simulink model "ball_and_plate"  (Simulink 7.6)
settings: Solver=ode45  StartTime=0.0  StopTime=20.0  RelTol=1e-3
undefined symbols (not defined in the file): magnitude
libraries: simulink x15
settings Model: Creator=Marco  LastModifiedBy=Marco

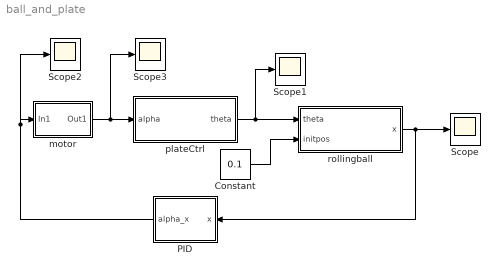
== system ball_and_plate ==
  Constant : Constant  Value=0.1
  PID : Subsystem
  Scope{,1..3} (4 alike) : Scope
      Scope settings: TimeRange=20  YMin=-2.5e+033  YMax=7e+033
      Scope2 settings: SaveName=ScopeData3
      Scope3 settings: SaveName=ScopeData4
  motor : Subsystem
  plateCtrl : Subsystem
  rollingball : Subsystem
  wires:
  plateCtrl/1(theta) -> rollingball/1(theta), Scope1/1
  rollingball/1(x) -> Scope/1, PID/1(x)
  Constant/1 -> rollingball/2(initpos)
  PID/1(alpha_x) -> motor/1(In1), Scope2/1
  motor/1(Out1) -> plateCtrl/1(alpha), Scope3/1

== system ball_and_plate/PID ==
  x : Inport
  controller : Subsystem
  alpha_x : Outport
  wires:
  controller/1(Out1) -> alpha_x/1
  x/1 -> controller/1(x)

== system ball_and_plate/motor ==
  In1 : Inport
  Rate Limiter : RateLimiter  RisingSlewLimit=7  FallingSlewLimit=-7  SampleTimeMode=inherited
  Out1 : Outport
  wires:
  In1/1 -> Rate Limiter/1
  Rate Limiter/1 -> Out1/1

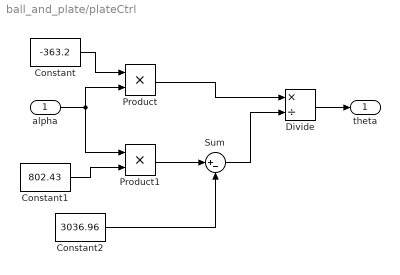
== system ball_and_plate/plateCtrl ==
  alpha : Inport
  Constant : Constant  Value=-363.2
  Constant1 : Constant  Value=802.43
  Constant2 : Constant  Value=3036.96
  Divide : Product  Inputs=*/
  Product : Product  RndMeth=Zero
  Product1 : Product  RndMeth=Zero
  Sum : Sum  Inputs=|+-
  theta : Outport
  wires:
  Constant/1 -> Product/1
  alpha/1 -> Product/2, Product1/1
  Constant1/1 -> Product1/2
  Product1/1 -> Sum/1
  Constant2/1 -> Sum/2
  Divide/1 -> theta/1
  Product/1 -> Divide/1
  Sum/1 -> Divide/2

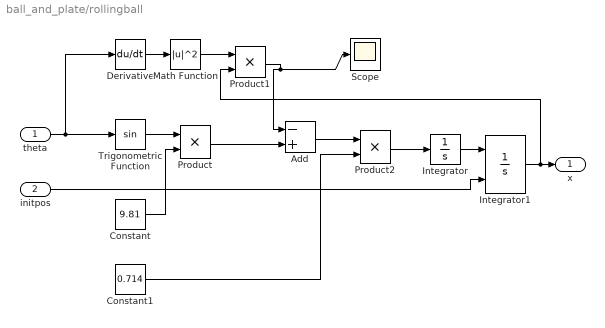
== system ball_and_plate/rollingball ==
  theta : Inport
  initpos : Inport  Port=2
  Add : Sum  Inputs=-+
  Constant : Constant  Value=9.81
  Constant1 : Constant  Value=0.714
  Derivative : Derivative
  Integrator : Integrator
  Integrator1 : Integrator  InitialConditionSource=external
  Math Function : Math  Operator=magnitude^2  SaturateOnIntegerOverflow=on
  Product : Product  RndMeth=Zero
  Product1 : Product  RndMeth=Zero
  Product2 : Product  RndMeth=Zero
  Scope : Scope
      settings: SaveName=ScopeData2
  Trigonometric Function : Trigonometry
  x : Outport
  wires:
  theta/1 -> Trigonometric Function/1, Derivative/1
  Trigonometric Function/1 -> Product/1
  Constant/1 -> Product/2
  Integrator/1 -> Integrator1/1
  Integrator1/1 -> Product1/2, x/1
  initpos/1 -> Integrator1/2
  Derivative/1 -> Math Function/1
  Math Function/1 -> Product1/1
  Product2/1 -> Integrator/1
  Constant1/1 -> Product2/2
  Add/1 -> Product2/1
  Product/1 -> Add/2
  Product1/1 -> Scope/1, Add/1

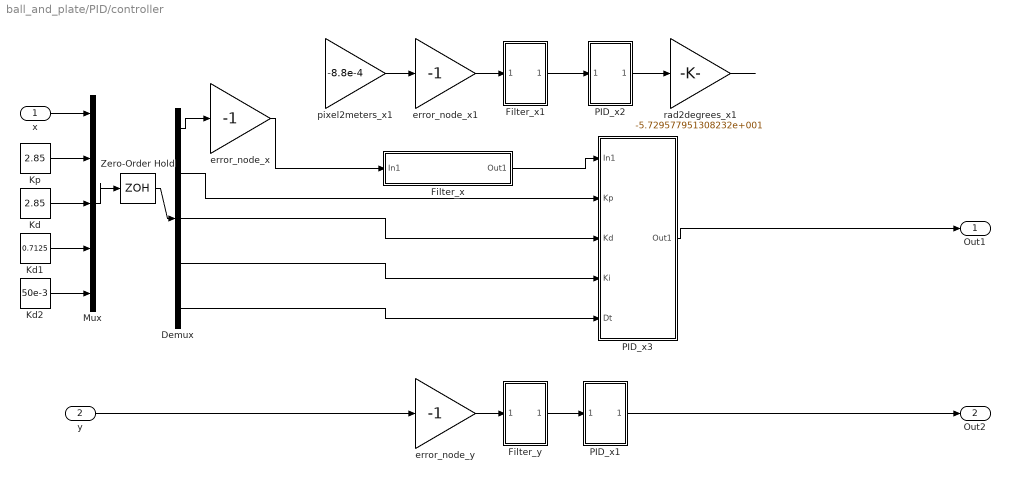
== system ball_and_plate/PID/controller ==
  x : Inport
  y : Inport  Port=2
  Demux : Demux  Outputs=5
  Filter_x : Subsystem
  Filter_x1 : Subsystem
  Filter_y : Subsystem
  Kd : Constant  Value=2.85  SampleTime=0
  Kd1 : Constant  Value=0.7125  SampleTime=0
  Kd2 : Constant  Value=50e-3  SampleTime=0
  Kp : Constant  Value=2.85  SampleTime=0
  Mux : Mux  Inputs=5
  PID_x1 : Subsystem
  PID_x2 : Subsystem
  PID_x3 : Subsystem
  Zero-Order Hold : ZeroOrderHold  SampleTime=50e-3
  error_node_x : Gain  Gain=-1
  error_node_x1 : Gain  Gain=-1
  error_node_y : Gain  Gain=-1  SampleTime=50e-3
  pixel2meters_x1 : Gain  Gain=-8.8e-4
  rad2degrees_x1 : Gain  Gain=-5.729577951308232e+001  SampleTime=50e-3
  Out1 : Outport
  Out2 : Outport  Port=2
  wires:
  PID_x1/1(Out1) -> Out2/1
  y/1 -> error_node_y/1
  Filter_x1/1(Out1) -> PID_x2/1(In1)
  rad2degrees_x1/1 -> ?
  error_node_x1/1 -> Filter_x1/1(In1)
  ? -> pixel2meters_x1/1
  pixel2meters_x1/1 -> error_node_x1/1
  PID_x2/1(Out1) -> rad2degrees_x1/1
  PID_x3/1(Out1) -> Out1/1
  error_node_y/1 -> Filter_y/1(In1)
  Filter_y/1(Out1) -> PID_x1/1(In1)
  error_node_x/1 -> Filter_x/1(In1)
  Filter_x/1(Out1) -> PID_x3/1(In1)
  x/1 -> Mux/1
  Mux/1 -> Zero-Order Hold/1
  Zero-Order Hold/1 -> Demux/1
  Demux/1 -> error_node_x/1
  Kd/1 -> Mux/3
  Kd1/1 -> Mux/4
  Demux/3 -> PID_x3/3(Kd)
  Demux/4 -> PID_x3/4(Ki)
  Kd2/1 -> Mux/5
  Demux/5 -> PID_x3/5(Dt)
  Kp/1 -> Mux/2
  Demux/2 -> PID_x3/2(Kp)

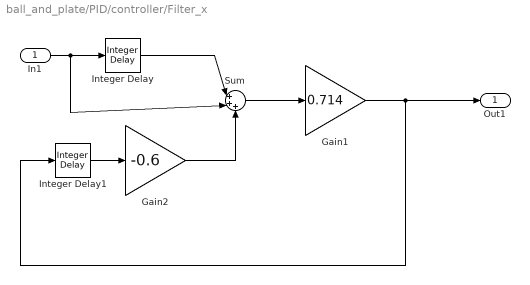
== system ball_and_plate/PID/controller/Filter_x ==
  In1 : Inport
  Gain1 : Gain  Gain=0.714
  Gain2 : Gain  Gain=-0.6
  Integer Delay : simulink/Discrete/Integer Delay  NumDelays=1  InputProcessing=Inherited  vinit=0.0  samptime=-1
  Integer Delay1 : simulink/Discrete/Integer Delay  NumDelays=1  InputProcessing=Inherited  vinit=0.0  samptime=-1
  Sum : Sum  Inputs=|+++
  Out1 : Outport
  wires:
  Sum/1 -> Gain1/1
  Gain1/1 -> Integer Delay1/1, Out1/1
  Integer Delay1/1 -> Gain2/1
  Integer Delay/1 -> Sum/1
  Gain2/1 -> Sum/3
  In1/1 -> Integer Delay/1, Sum/2

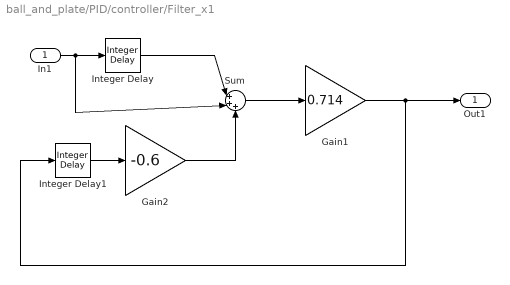
== system ball_and_plate/PID/controller/Filter_x1 ==
  In1 : Inport
  Gain1 : Gain  Gain=0.714  SampleTime=50e-3
  Gain2 : Gain  Gain=-0.6  SampleTime=50e-3
  Integer Delay : simulink/Discrete/Integer Delay  NumDelays=1  InputProcessing=Inherited  vinit=0.0  samptime=-1
  Integer Delay1 : simulink/Discrete/Integer Delay  NumDelays=1  InputProcessing=Inherited  vinit=0.0  samptime=50e-3
  Sum : Sum  Inputs=|+++  SampleTime=50e-3
  Out1 : Outport
  wires:
  In1/1 -> Integer Delay/1, Sum/2
  Sum/1 -> Gain1/1
  Gain1/1 -> Out1/1, Integer Delay1/1
  Integer Delay1/1 -> Gain2/1
  Integer Delay/1 -> Sum/1
  Gain2/1 -> Sum/3

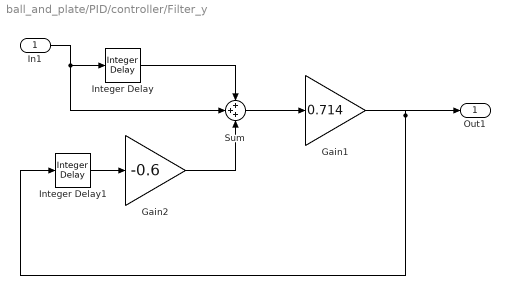
== system ball_and_plate/PID/controller/Filter_y ==
  In1 : Inport
  Gain1 : Gain  Gain=0.714  SampleTime=50e-3
  Gain2 : Gain  Gain=-0.6  SampleTime=50e-3
  Integer Delay : simulink/Discrete/Integer Delay  NumDelays=1  InputProcessing=Inherited  vinit=0.0  samptime=50e-3
  Integer Delay1 : simulink/Discrete/Integer Delay  NumDelays=1  InputProcessing=Inherited  vinit=0.0  samptime=50e-3
  Sum : Sum  Inputs=+++  SampleTime=50e-3
  Out1 : Outport
  wires:
  Integer Delay1/1 -> Gain2/1
  Gain1/1 -> Integer Delay1/1, Out1/1
  Sum/1 -> Gain1/1
  Integer Delay/1 -> Sum/1
  In1/1 -> Integer Delay/1, Sum/2
  Gain2/1 -> Sum/3

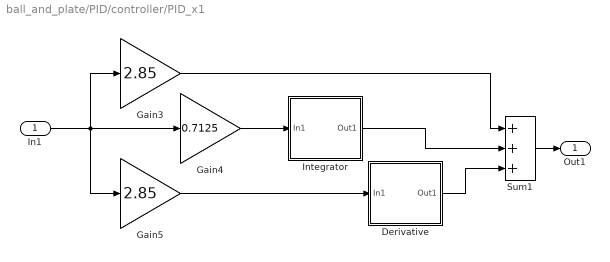
== system ball_and_plate/PID/controller/PID_x1 ==
  In1 : Inport
  Derivative : Subsystem
  Gain3 : Gain  Gain=2.85  SampleTime=50e-3
  Gain4 : Gain  Gain=0.7125  SampleTime=50e-3
  Gain5 : Gain  Gain=2.85  SampleTime=50e-3
  Integrator : Subsystem
  Sum1 : Sum  Inputs=+++  SampleTime=50e-3
  Out1 : Outport
  wires:
  Sum1/1 -> Out1/1
  Gain5/1 -> Derivative/1(In1)
  Gain4/1 -> Integrator/1(In1)
  Gain3/1 -> Sum1/1
  In1/1 -> Gain5/1, Gain3/1, Gain4/1
  Integrator/1(Out1) -> Sum1/2
  Derivative/1(Out1) -> Sum1/3

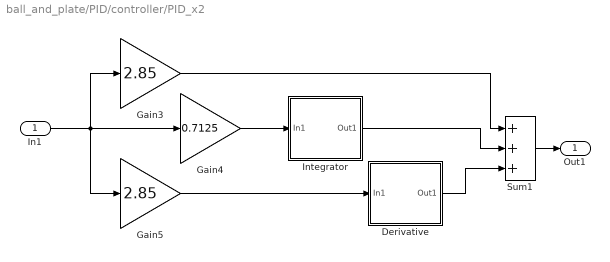
== system ball_and_plate/PID/controller/PID_x2 ==
  In1 : Inport
  Derivative : Subsystem
  Gain3 : Gain  Gain=2.85  SampleTime=50e-3
  Gain4 : Gain  Gain=0.7125  SampleTime=50e-3
  Gain5 : Gain  Gain=2.85  SampleTime=50e-3
  Integrator : Subsystem
  Sum1 : Sum  Inputs=+++  SampleTime=50e-3
  Out1 : Outport
  wires:
  In1/1 -> Gain4/1, Gain3/1, Gain5/1
  Gain3/1 -> Sum1/1
  Gain4/1 -> Integrator/1(In1)
  Gain5/1 -> Derivative/1(In1)
  Derivative/1(Out1) -> Sum1/3
  Integrator/1(Out1) -> Sum1/2
  Sum1/1 -> Out1/1

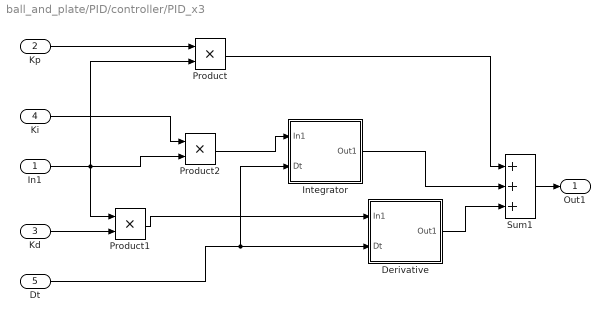
== system ball_and_plate/PID/controller/PID_x3 ==
  In1 : Inport
  Kp : Inport  Port=2
  Kd : Inport  Port=3
  Ki : Inport  Port=4
  Dt : Inport  Port=5
  Derivative : Subsystem
  Integrator : Subsystem
  Product : Product  RndMeth=Zero
  Product1 : Product  RndMeth=Zero
  Product2 : Product  RndMeth=Zero
  Sum1 : Sum  Inputs=+++
  Out1 : Outport
  wires:
  Sum1/1 -> Out1/1
  Product1/1 -> Derivative/1(In1)
  Product2/1 -> Integrator/1(In1)
  Product/1 -> Sum1/1
  In1/1 -> Product/2, Product1/1, Product2/2
  Integrator/1(Out1) -> Sum1/2
  Derivative/1(Out1) -> Sum1/3
  Kp/1 -> Product/1
  Kd/1 -> Product1/2
  Ki/1 -> Product2/1
  Dt/1 -> Derivative/2(Dt), Integrator/2(Dt)

== system ball_and_plate/PID/controller/PID_x1/Derivative ==
  In1 : Inport
  Gain3 : Gain  Gain=20  SampleTime=50e-3
  Integer Delay1 : simulink/Discrete/Integer Delay  NumDelays=1  InputProcessing=Inherited  vinit=0.0  samptime=50e-3
  Sum : Sum  Inputs=|+-
  Out1 : Outport
  wires:
  Gain3/1 -> Out1/1
  In1/1 -> Sum/1, Integer Delay1/1
  Sum/1 -> Gain3/1
  Integer Delay1/1 -> Sum/2

== system ball_and_plate/PID/controller/PID_x1/Integrator ==
  In1 : Inport
  Gain1 : Gain  Gain=50e-3  SampleTime=50e-3
  Integer Delay : simulink/Discrete/Integer Delay  NumDelays=1  InputProcessing=Inherited  vinit=0.0  samptime=50e-3
  Integer Delay1 : simulink/Discrete/Integer Delay  NumDelays=1  InputProcessing=Inherited  vinit=0.0  samptime=50e-3
  Sum : Sum  Inputs=|++
  Out1 : Outport
  wires:
  Gain1/1 -> Sum/1
  Integer Delay/1 -> Gain1/1
  Sum/1 -> Integer Delay1/1, Out1/1
  In1/1 -> Integer Delay/1
  Integer Delay1/1 -> Sum/2

== system ball_and_plate/PID/controller/PID_x2/Derivative ==
  In1 : Inport
  Gain3 : Gain  Gain=20  SampleTime=50e-3
  Integer Delay1 : simulink/Discrete/Integer Delay  NumDelays=1  InputProcessing=Inherited  vinit=0.0  samptime=50e-3
  Sum : Sum  Inputs=|+-
  Out1 : Outport
  wires:
  Integer Delay1/1 -> Sum/2
  Sum/1 -> Gain3/1
  In1/1 -> Integer Delay1/1, Sum/1
  Gain3/1 -> Out1/1

== system ball_and_plate/PID/controller/PID_x2/Integrator ==
  In1 : Inport
  Gain1 : Gain  Gain=50e-3  SampleTime=50e-3
  Integer Delay : simulink/Discrete/Integer Delay  NumDelays=1  InputProcessing=Inherited  vinit=0.0  samptime=50e-3
  Integer Delay1 : simulink/Discrete/Integer Delay  NumDelays=1  InputProcessing=Inherited  vinit=0.0  samptime=50e-3
  Sum : Sum  Inputs=|++
  Out1 : Outport
  wires:
  Integer Delay1/1 -> Sum/2
  In1/1 -> Integer Delay/1
  Sum/1 -> Out1/1, Integer Delay1/1
  Integer Delay/1 -> Gain1/1
  Gain1/1 -> Sum/1

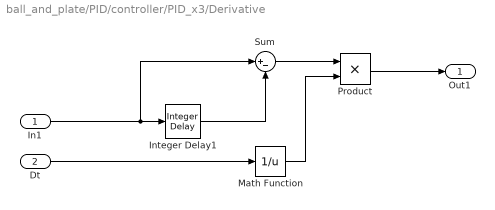
== system ball_and_plate/PID/controller/PID_x3/Derivative ==
  In1 : Inport
  Dt : Inport  Port=2
  Integer Delay1 : simulink/Discrete/Integer Delay  NumDelays=1  InputProcessing=Inherited  vinit=0.0  samptime=-1
  Math Function : Math  Operator=reciprocal  SaturateOnIntegerOverflow=on
  Product : Product  RndMeth=Zero
  Sum : Sum  Inputs=|+-
  Out1 : Outport
  wires:
  In1/1 -> Sum/1, Integer Delay1/1
  Sum/1 -> Product/1
  Integer Delay1/1 -> Sum/2
  Dt/1 -> Math Function/1
  Math Function/1 -> Product/2
  Product/1 -> Out1/1

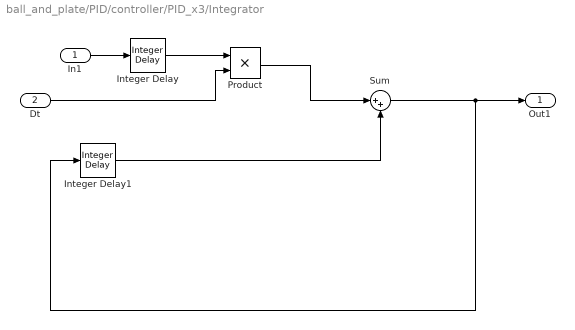
== system ball_and_plate/PID/controller/PID_x3/Integrator ==
  In1 : Inport
  Dt : Inport  Port=2
  Integer Delay : simulink/Discrete/Integer Delay  NumDelays=1  InputProcessing=Inherited  vinit=0.0  samptime=-1
  Integer Delay1 : simulink/Discrete/Integer Delay  NumDelays=1  InputProcessing=Inherited  vinit=0.0  samptime=-1
  Product : Product  RndMeth=Zero
  Sum : Sum  Inputs=|++
  Out1 : Outport
  wires:
  Product/1 -> Sum/1
  Integer Delay/1 -> Product/1
  Sum/1 -> Integer Delay1/1, Out1/1
  In1/1 -> Integer Delay/1
  Integer Delay1/1 -> Sum/2
  Dt/1 -> Product/2
